simulink model "OORT"  (Simulink 7.6)
settings: Solver=ode3  SolverMode=SingleTasking  StartTime=0.0  StopTime=1.2  FixedStep=2e-5  RelTol=1e-4  AbsTol=1e-6
undefined symbols (not defined in the file or in its folder): DAB, den, elements, num
libraries: powerlib x179, powerlib_extras x6
(part 1 of 4)
settings Model: Creator=azadpour  LastModifiedBy=PC  ExtModeTrigMode=oneshot  ExtModeArmWhenConnect=off
settings SolverCC: SolverResetMethod=Robust
settings DataIOCC: LimitDataPoints=off
settings OptimizationCC: BlockReduction=off  BooleanDataType=off  InlineInvariantSignals=on  InitFltsAndDblsToZero=on
settings DebuggingCC: SaveWithDisabledLinksMsg=none  SaveWithParameterizedLinksMsg=none  CheckSSInitialOutputMsg=off  SignalResolutionControl=TryResolveAllWithWarning  SolverPrmCheckMsg=none  InheritedTsInSrcMsg=none  DiscreteInheritContinuousMsg=none  MultiTaskDSMMsg=none  MultiTaskCondExecSysMsg=none  TasksWithSamePriorityMsg=none  SigSpecEnsureSampleTimeMsg=none  IntegerOverflowMsg=none  Int32ToFloatConvMsg=none  ParameterPrecisionLossMsg=none  ParameterTunabilityLossMsg=none  UnconnectedInputMsg=none  UnconnectedOutputMsg=none  UnconnectedLineMsg=none  BusObjectLabelMismatch=none  RootOutportRequireBusObject=none  ModelReferenceDataLoggingMessage=none  StrictBusMsg=None
settings HardwareCC: TargetHWDeviceType=32-bit Generic  TargetUnknown=on  ProdEqTarget=off
settings GRTTargetCC: TargetFcnLib=ansi_tfl_tmw.mat

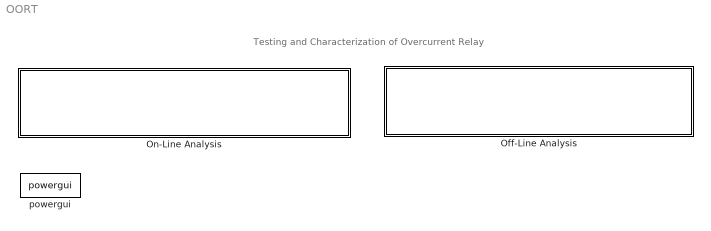
== system OORT ==
  note: Testing and Characterization of Overcurrent Relay
  Off-Line Analysis : Subsystem
      mask Type: Off-Line Analysis
      mask Display: disp('Off-Line Testing');
  On-Line Analysis : Subsystem
      mask Type: On-Line Analysis
      mask Display: disp('On-Line Testing')
  powergui : powerlib/powergui  SystemSampleTime=-1  SimulationMode=Continuous  SampleTime=0  frequency=60  SPID=off  DisableSnubberDevices=off  DisableRonSwitches=off  DisableVfSwitches=off  SwTol=0  Interpol=off  frequencyindice=60  echomessages=off  HookPort=off  DisplayEquations=off  FunctionMessages=off  EnableUseOfTLC=off  x0status=blocks  RestoreLinks=warning  ResistiveCurrentMeasurement=off  Frange=[0:2:500]  Ylog=off  Xlog=on  ShowGrid=off  save=off  variable=ZData  ZoomFFT=on  StartTime=0.0  cycles=1  DisplayStyle=1  fundamental=60  FreqAxis=off  MaxFrequency=1000  frequencyindicesteady=1  RmsSteady=1  display=off  Ts=0  methode=off

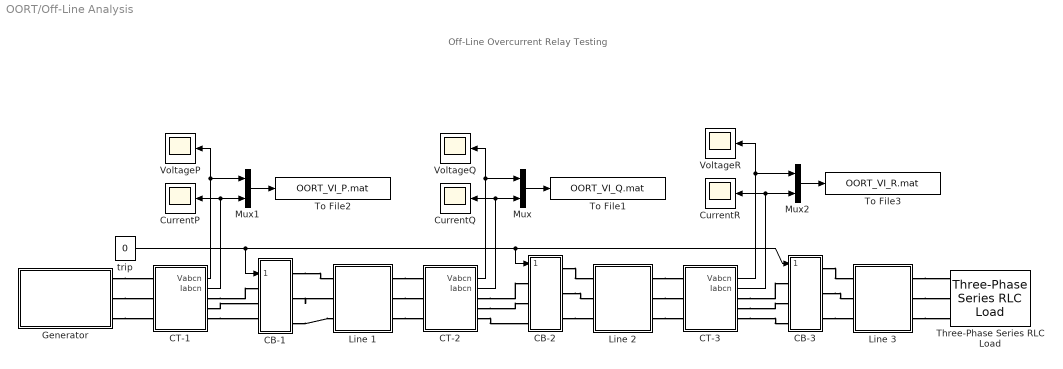
== system OORT/Off-Line Analysis ==
  note: Off-Line Overcurrent Relay Testing
  CB-1 : Subsystem  mask{t_op=0.02}
      mask prompts: t_op "Operating time [s]"
  CB-2 : Subsystem  mask{t_op=0.02}
      mask prompts: t_op "Operating time [s]"
  CB-3 : Subsystem  mask{t_op=0.02}
      mask prompts: t_op "Operating time [s]"
  CT-1 : Subsystem  mask{VT=2000, CT=100}
      mask prompts: VT "VT ratio"; CT "CT ratio"
  CT-2 : Subsystem  mask{VT=2000, CT=100}
      mask prompts: VT "VT ratio"; CT "CT ratio"
  CT-3 : Subsystem  mask{VT=2000, CT=100}
      mask prompts: VT "VT ratio"; CT "CT ratio"
  CurrentP : Scope
      settings: TickLabels=on  YMin=-8000  YMax=9000  SaveName=ScopeData12  DataFormat=Array
  CurrentQ : Scope
      settings: TickLabels=on  YMin=-8000  YMax=9000  SaveName=ScopeData13  DataFormat=Array
  CurrentR : Scope
      settings: TickLabels=on  YMin=-8000  YMax=9000  SaveName=ScopeData14  DataFormat=Array
  Generator : Subsystem  mask(3-phase inductive source - Ungrounded neutral){V=194367, Phi=0, F=60, R=3.4878, L=0.1323}
      mask prompts: V "Voltage magnitude (V) :"; Phi "Phase angle of phase A (Degrees) :"; F "Frequency (Hz) :"; R "Source resistance (Ohms):"; L "Source inductance (H) :"
      mask init:
      | a=R;b=L;c=inf;
      | short_x =[0,150];
      | short_y =[0,0];
      | 
      | resistor_x = [0 30,30,38,53,68,83,98,113,120,120,150];
      | resistor_y = [0,0,0,25,-25,25,-25,25,-25,0,0,0];
      | 
      | inductor_x = [150,173,173,174,178,184,190,197,202,205,206,204,201,201,197,196,198,201,207,214,220,225,229,229,227,224,224,220,219,221,225,230,237,243,249,252,253,251,247,247,244,243,244,248,254,260,267,272,275,276,276,300];
      | 
      | inductor_y = [0,0,1,11,19,24,25,23,17,8,-2,-12,-18,-18,-9,1,11,19,24,25,23,17,8,-2,-12,-18,-18,-9,1,11,19,24,25,23,17,8,-2,-12,-18,-18,-9,1, 11,19,24,25,23,17,8,0,0,0];
      | 
      | capacitor_x1 = [300 360 360 360];
      | capacitor_y1 = [0 0 25 -25];
      | capacitor_x2 = [390 390 390 450];
      | capacitor_y2 = [25,-25,0,0];
      | if a~=0
      | 	s1=resistor_x;
      | 	s2=resistor_y;
      | else
      | 	s1=short_x;
      | 	s2=short_y;
      | end
      | 
      | if b~=0
      | 	s3=inductor_x;
      | 	s4=inductor_y;
      | else
      | 	s3=short_x+150;
      | 	s4=short_y;
      | end
      | 
      | s5=[];
      | s6=[];
      | s7=[];
      | s8=[];
      mask Display: plot(-170,-60,360,60,s1,s2,s3,s4,s5,s6,s7,s8, [0,9,18,24,29,30,29,24,18,9,0,-9,-18,-24,-29,-30,-29,-24,-18,-9,0]*1.5-45,  [30,29,24,18,9,0,-9,-18,-24,-29,-30,-29,-24,-18,-9,0,9,18,24,29,30]*0.8,[-150,-90],[0,0],[-150,-150],[-20,20],[-165,-165],[-15,15],[-180,-180],[-10,10])
  Line 1 : Subsystem  mask(Teansmission line with fault){ff=60, rr=[0.0815 0.3666], ll=[2.1e-3 6.5e-3], cc=[31.6e-9 12.7e-9], length=40, faultLocation=0.5, faultType='C-A-G', faultR=0.01, faultTime=[9 10 11 12 13]}
      mask prompts: ff "Frequency used for R L C specification (Hz)"; rr "Resistance per unit length (Ohm/mile) [R1 R0]"; ll "Inductance per unit length (H/mile) [L1 L0]"; cc "Capacitance per unit length (F/mile) [C1 C0]"; length "Line length (mile)"; faultLocation "Fault location (p.u.) <0,1>"; faultType "Fault Type"; faultR "Fault Resistance per Phase (Ohm)"; faultTime "Fault time sequence (s) [C O C O C]"
      mask StyleString: edit,edit,edit,edit,edit,edit,popup('A-G'|'B-G'|'C-G'|'B-C'|'B-C-G'|'C-A'|'C-A-G'|'A-B-C'|'A-B-C-G'),edit,edit
  Line 2 : Subsystem  mask(Teansmission line with fault){ff=60, rr=[0.0815 0.3666], ll=[2.1e-3 6.5e-3], cc=[31.6e-9 12.7e-9], length=40, faultLocation=0.5, faultType='C-A-G', faultR=0.01, faultTime=[9 10 11 12 13]}
      mask prompts: ff "Frequency used for R L C specification (Hz)"; rr "Resistance per unit length (Ohm/mile) [R1 R0]"; ll "Inductance per unit length (H/mile) [L1 L0]"; cc "Capacitance per unit length (F/mile) [C1 C0]"; length "Line length (mile)"; faultLocation "Fault location (p.u.) <0,1>"; faultType "Fault Type"; faultR "Fault Resistance per Phase (Ohm)"; faultTime "Fault time sequence (s) [C O C O C]"
      mask StyleString: edit,edit,edit,edit,edit,edit,popup('A-G'|'B-G'|'C-G'|'B-C'|'B-C-G'|'C-A'|'C-A-G'|'A-B-C'|'A-B-C-G'),edit,edit
  Line 3 : Subsystem  mask(Teansmission line with fault){ff=60, rr=[0.0815 0.3666], ll=[2.1e-3 6.5e-3], cc=[31.6e-9 12.7e-9], length=40, faultLocation=0.9, faultType='A-B-C', faultR=0.01, faultTime=[0.02 10 11 12 13]}
      mask prompts: ff "Frequency used for R L C specification (Hz)"; rr "Resistance per unit length (Ohm/mile) [R1 R0]"; ll "Inductance per unit length (H/mile) [L1 L0]"; cc "Capacitance per unit length (F/mile) [C1 C0]"; length "Line length (mile)"; faultLocation "Fault location (p.u.) <0,1>"; faultType "Fault Type"; faultR "Fault Resistance per Phase (Ohm)"; faultTime "Fault time sequence (s) [C O C O C]"
      mask StyleString: edit,edit,edit,edit,edit,edit,popup('A-G'|'B-G'|'C-G'|'B-C'|'B-C-G'|'C-A'|'C-A-G'|'A-B-C'|'A-B-C-G'),edit,edit
  Mux : Mux  Inputs=2
  Mux1 : Mux  Inputs=2
  Mux2 : Mux  Inputs=2
  Three-Phase Series RLC Load : powerlib/Elements/Three-Phase Series RLC Load  DialogController=POWERSYS.PowerSysDialog  PhysicalDomain=powersysdomain  SubClassName=unknown  LeftPortType=p1  RightPortType=p1  LConnTagsString=A|B|C  Configuration=Y (grounded)  NominalVoltage=230e3  NominalFrequency=60  ActivePower=54e3  InductivePower=26e3  CapacitivePower=0  Measurements=None
  To File1 : ToFile  Filename=OORT_VI_Q.mat
  To File2 : ToFile  Filename=OORT_VI_P.mat
  To File3 : ToFile  Filename=OORT_VI_R.mat
  VoltageP : Scope
      settings: TickLabels=on  YMin=-8000  YMax=9000  SaveName=ScopeData21  DataFormat=Array
  VoltageQ : Scope
      settings: TickLabels=on  YMin=-8000  YMax=9000  SaveName=ScopeData22  DataFormat=Array
  VoltageR : Scope
      settings: TickLabels=on  YMin=-8000  YMax=9000  SaveName=ScopeData23  DataFormat=Array
  trip : Constant  Value=0
  wires:
  CT-2/2(Iabcn) -> CurrentQ/1, Mux/2
  CT-2/1(Vabcn) -> VoltageQ/1, Mux/1
  CT-1/2(Iabcn) -> CurrentP/1, Mux1/2
  CT-1/1(Vabcn) -> VoltageP/1, Mux1/1
  CT-3/2(Iabcn) -> CurrentR/1, Mux2/2
  CT-3/1(Vabcn) -> VoltageR/1, Mux2/1
  Mux/1 -> To File1/1
  Mux1/1 -> To File2/1
  Mux2/1 -> To File3/1
  trip/1 -> CB-1/1(Trip), CB-2/1(Trip), CB-3/1(Trip)
  connections:
  Line 1/RConn1 -- CT-2/LConn1
  Line 1/RConn2 -- CT-2/LConn2
  Line 1/RConn3 -- CT-2/LConn3
  Generator/RConn1 -- CT-1/LConn1
  Generator/RConn2 -- CT-1/LConn2
  Generator/RConn3 -- CT-1/LConn3
  CT-1/RConn1 -- CB-1/LConn1
  CT-1/RConn2 -- CB-1/LConn2
  CT-1/RConn3 -- CB-1/LConn3
  CB-1/RConn1 -- Line 1/LConn1
  CB-1/RConn2 -- Line 1/LConn2
  CB-1/RConn3 -- Line 1/LConn3
  CT-2/RConn1 -- CB-2/LConn1
  CT-2/RConn2 -- CB-2/LConn2
  CT-2/RConn3 -- CB-2/LConn3
  CB-2/RConn1 -- Line 2/LConn1
  CB-2/RConn2 -- Line 2/LConn2
  CB-2/RConn3 -- Line 2/LConn3
  Line 2/RConn1 -- CT-3/LConn1
  Line 2/RConn2 -- CT-3/LConn2
  Line 2/RConn3 -- CT-3/LConn3
  CT-3/RConn1 -- CB-3/LConn1
  CT-3/RConn2 -- CB-3/LConn2
  CT-3/RConn3 -- CB-3/LConn3
  CB-3/RConn1 -- Line 3/LConn1
  CB-3/RConn2 -- Line 3/LConn2
  CB-3/RConn3 -- Line 3/LConn3
  Line 3/RConn1 -- Three-Phase Series RLC Load/LConn1
  Line 3/RConn2 -- Three-Phase Series RLC Load/LConn2
  Line 3/RConn3 -- Three-Phase Series RLC Load/LConn3

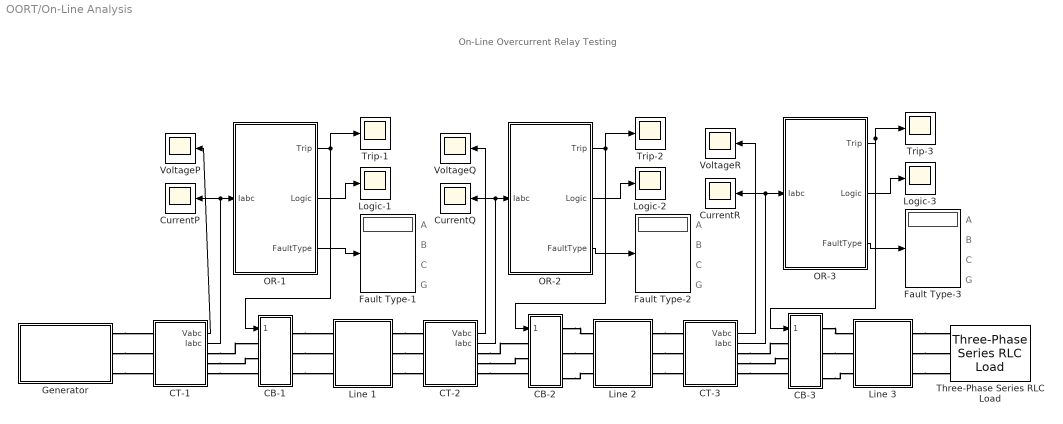
== system OORT/On-Line Analysis ==
  note: On-Line Overcurrent Relay Testing
  note: A
  note: B
  note: C
  note: G
  note: A
  note: B
  note: C
  note: G
  note: A
  note: B
  note: C
  note: G
  CB-1 : Subsystem  mask{t_op=0.02}
      mask prompts: t_op "Operating time [s]"
  CB-2 : Subsystem  mask{t_op=0.02}
      mask prompts: t_op "Operating time [s]"
  CB-3 : Subsystem  mask{t_op=0.02}
      mask prompts: t_op "Operating time [s]"
  CT-1 : Subsystem  mask{VT=2000, CT=100}
      mask prompts: VT "VT ratio"; CT "CT ratio"
  CT-2 : Subsystem  mask{VT=2000, CT=100}
      mask prompts: VT "VT ratio"; CT "CT ratio"
  CT-3 : Subsystem  mask{VT=2000, CT=100}
      mask prompts: VT "VT ratio"; CT "CT ratio"
  CurrentP : Scope
      settings: TickLabels=on  YMin=-8000  YMax=9000  SaveName=ScopeData2  DataFormat=Array
  CurrentQ : Scope
      settings: TickLabels=on  YMin=-8000  YMax=9000  DataFormat=Array
  CurrentR : Scope
      settings: TickLabels=on  YMin=-8000  YMax=9000  SaveName=ScopeData8  DataFormat=Array
  Fault Type-1 : Display
  Fault Type-2 : Display
  Fault Type-3 : Display
  Generator : Subsystem  mask(3-phase inductive source - Ungrounded neutral){V=194367, Phi=0, F=60, R=3.4878, L=0.1323}
      mask prompts: V "Voltage magnitude (V) :"; Phi "Phase angle of phase A (Degrees) :"; F "Frequency (Hz) :"; R "Source resistance (Ohms):"; L "Source inductance (H) :"
      mask init: same as OORT/Off-Line Analysis/Generator
      mask Display: plot(-170,-60,360,60,s1,s2,s3,s4,s5,s6,s7,s8, [0,9,18,24,29,30,29,24,18,9,0,-9,-18,-24,-29,-30,-29,-24,-18,-9,0]*1.5-45,  [30,29,24,18,9,0,-9,-18,-24,-29,-30,-29,-24,-18,-9,0,9,18,24,29,30]*0.8,[-150,-90],[0,0],[-150,-150],[-20,20],[-165,-165],[-15,15],[-180,-180],[-10,10])
  Line 1 : Subsystem  mask(Teansmission line with fault){ff=60, rr=[0.0815 0.3666], ll=[2.1e-3 6.5e-3], cc=[31.6e-9 12.7e-9], length=40, faultLocation=0.5, faultType='C-A-G', faultR=0.01, faultTime=[9 10 11 12 13]}
      mask prompts: ff "Frequency used for R L C specification (Hz)"; rr "Resistance per unit length (Ohm/mile) [R1 R0]"; ll "Inductance per unit length (H/mile) [L1 L0]"; cc "Capacitance per unit length (F/mile) [C1 C0]"; length "Line length (mile)"; faultLocation "Fault location (p.u.) <0,1>"; faultType "Fault Type"; faultR "Fault Resistance per Phase (Ohm)"; faultTime "Fault time sequence (s) [C O C O C]"
      mask StyleString: edit,edit,edit,edit,edit,edit,popup('A-G'|'B-G'|'C-G'|'B-C'|'B-C-G'|'C-A'|'C-A-G'|'A-B-C'|'A-B-C-G'),edit,edit
  Line 2 : Subsystem  mask(Teansmission line with fault){ff=60, rr=[0.0815 0.3666], ll=[2.1e-3 6.5e-3], cc=[31.6e-9 12.7e-9], length=40, faultLocation=0.3, faultType='B-C', faultR=0.01, faultTime=[9 10 11 12 13]}
      mask prompts: ff "Frequency used for R L C specification (Hz)"; rr "Resistance per unit length (Ohm/mile) [R1 R0]"; ll "Inductance per unit length (H/mile) [L1 L0]"; cc "Capacitance per unit length (F/mile) [C1 C0]"; length "Line length (mile)"; faultLocation "Fault location (p.u.) <0,1>"; faultType "Fault Type"; faultR "Fault Resistance per Phase (Ohm)"; faultTime "Fault time sequence (s) [C O C O C]"
      mask StyleString: edit,edit,edit,edit,edit,edit,popup('A-G'|'B-G'|'C-G'|'B-C'|'B-C-G'|'C-A'|'C-A-G'|'A-B-C'|'A-B-C-G'),edit,edit
  Line 3 : Subsystem  mask(Teansmission line with fault){ff=60, rr=[0.0815 0.3666], ll=[2.1e-3 6.5e-3], cc=[31.6e-9 12.7e-9], length=40, faultLocation=0.9, faultType='A-B-C', faultR=0.01, faultTime=[0.02 10 11 12 13]}
      mask prompts: ff "Frequency used for R L C specification (Hz)"; rr "Resistance per unit length (Ohm/mile) [R1 R0]"; ll "Inductance per unit length (H/mile) [L1 L0]"; cc "Capacitance per unit length (F/mile) [C1 C0]"; length "Line length (mile)"; faultLocation "Fault location (p.u.) <0,1>"; faultType "Fault Type"; faultR "Fault Resistance per Phase (Ohm)"; faultTime "Fault time sequence (s) [C O C O C]"
      mask StyleString: edit,edit,edit,edit,edit,edit,popup('A-G'|'B-G'|'C-G'|'B-C'|'B-C-G'|'C-A'|'C-A-G'|'A-B-C'|'A-B-C-G'),edit,edit
  Logic-1 : Scope
      settings: SaveName=ScopeData3
  Logic-2 : Scope
      settings: SaveName=ScopeData7
  Logic-3 : Scope
      settings: SaveName=ScopeData9
  OR-1 : Subsystem  mask(Overcurrent Relay){Iop=3.8, Td=1, ResCurr=0.1}
      mask prompts: Iop "Pickup Current (A):"; Td "Time Delay (s):"; ResCurr "ResidualCurrent Threshold (A):"
  OR-2 : Subsystem  mask(Overcurrent Relay){Iop=2.6, Td=0.6, ResCurr=0.1}
      mask prompts: Iop "Pickup Current (A):"; Td "Time Delay (s):"; ResCurr "ResidualCurrent Threshold (A):"
  OR-3 : Subsystem  mask(Overcurrent Relay){Iop=1.4, Td=0, ResCurr=0.1}
      mask prompts: Iop "Pickup Current (A):"; Td "Time Delay (s):"; ResCurr "ResidualCurrent Threshold (A):"
  Three-Phase Series RLC Load : powerlib/Elements/Three-Phase Series RLC Load  DialogController=POWERSYS.PowerSysDialog  PhysicalDomain=powersysdomain  SubClassName=unknown  LeftPortType=p1  RightPortType=p1  LConnTagsString=A|B|C  Configuration=Y (grounded)  NominalVoltage=230e3  NominalFrequency=60  ActivePower=54e3  InductivePower=26e3  CapacitivePower=0  Measurements=None
  Trip-1 : Scope
      settings: YMin=-0.2  YMax=1.2  SaveName=ScopeData4
  Trip-2 : Scope
      settings: YMin=-0.2  YMax=1.2  SaveName=ScopeData6
  Trip-3 : Scope
      settings: TimeRange=0.2  YMin=-0.2  YMax=1.2  SaveName=ScopeData10
  VoltageP : Scope
      settings: TickLabels=on  YMin=-8000  YMax=9000  SaveName=ScopeData5  DataFormat=Array
  VoltageQ : Scope
      settings: TickLabels=on  YMin=-8000  YMax=9000  DataFormat=Array
  VoltageR : Scope
      settings: TickLabels=on  YMin=-8000  YMax=9000  SaveName=ScopeData11  DataFormat=Array
  wires:
  CT-2/2(Iabc) -> CurrentQ/1, OR-2/1(Iabc)
  CT-2/1(Vabc) -> VoltageQ/1
  OR-2/1(Trip) -> Trip-2/1, CB-2/1(Trip)
  OR-2/2(Logic) -> Logic-2/1
  OR-2/3(FaultType) -> Fault Type-2/1
  OR-1/1(Trip) -> Trip-1/1, CB-1/1(Trip)
  OR-1/2(Logic) -> Logic-1/1
  CT-1/2(Iabc) -> OR-1/1(Iabc), CurrentP/1
  CT-1/1(Vabc) -> VoltageP/1
  OR-3/1(Trip) -> Trip-3/1, CB-3/1(Trip)
  OR-3/2(Logic) -> Logic-3/1
  OR-3/3(FaultType) -> Fault Type-3/1
  CT-3/2(Iabc) -> CurrentR/1, OR-3/1(Iabc)
  CT-3/1(Vabc) -> VoltageR/1
  OR-1/3(FaultType) -> Fault Type-1/1
  connections:
  Line 1/RConn1 -- CT-2/LConn1
  Line 1/RConn2 -- CT-2/LConn2
  Line 1/RConn3 -- CT-2/LConn3
  Generator/RConn1 -- CT-1/LConn1
  Generator/RConn2 -- CT-1/LConn2
  Generator/RConn3 -- CT-1/LConn3
  CT-1/RConn1 -- CB-1/LConn1
  CT-1/RConn2 -- CB-1/LConn2
  CT-1/RConn3 -- CB-1/LConn3
  CB-1/RConn1 -- Line 1/LConn1
  CB-1/RConn2 -- Line 1/LConn2
  CB-1/RConn3 -- Line 1/LConn3
  CT-2/RConn1 -- CB-2/LConn1
  CT-2/RConn2 -- CB-2/LConn2
  CT-2/RConn3 -- CB-2/LConn3
  CB-2/RConn1 -- Line 2/LConn1
  CB-2/RConn2 -- Line 2/LConn2
  CB-2/RConn3 -- Line 2/LConn3
  Line 2/RConn1 -- CT-3/LConn1
  Line 2/RConn2 -- CT-3/LConn2
  Line 2/RConn3 -- CT-3/LConn3
  CT-3/RConn1 -- CB-3/LConn1
  CT-3/RConn2 -- CB-3/LConn2
  CT-3/RConn3 -- CB-3/LConn3
  CB-3/RConn1 -- Line 3/LConn1
  CB-3/RConn2 -- Line 3/LConn2
  CB-3/RConn3 -- Line 3/LConn3
  Line 3/RConn1 -- Three-Phase Series RLC Load/LConn1
  Line 3/RConn2 -- Three-Phase Series RLC Load/LConn2
  Line 3/RConn3 -- Three-Phase Series RLC Load/LConn3

== system OORT/Off-Line Analysis/CB-1 ==
  Trip : Inport
  BreakerA : powerlib/Elements/Breaker  DialogController=POWERSYS.PowerSysDialog  SystemSampleTime=-1  BreakerResistance=0.01  InitialState=1  SnubberResistance=1e6  SnubberCapacitance=inf  SwitchingTimes="[ 1/60  5/60 ]"  External=on  Measurements=None  MoreParameters=off  NoBreakLoop=off
  BreakerB : powerlib/Elements/Breaker  DialogController=POWERSYS.PowerSysDialog  SystemSampleTime=-1  BreakerResistance=0.01  InitialState=1  SnubberResistance=1e6  SnubberCapacitance=inf  SwitchingTimes="[ 1/60  5/60 ]"  External=on  Measurements=None  MoreParameters=off  NoBreakLoop=off
  BreakerC : powerlib/Elements/Breaker  DialogController=POWERSYS.PowerSysDialog  SystemSampleTime=-1  BreakerResistance=0.01  InitialState=1  SnubberResistance=1e6  SnubberCapacitance=inf  SwitchingTimes="[ 1/60  5/60 ]"  External=on  Measurements=None  MoreParameters=off  NoBreakLoop=off
  NOT : Logic  Operator=NOT  Inputs=1
  Series RLC Branch1 : powerlib/Elements/Series RLC Branch  DialogController=POWERSYS.PowerSysDialog  PhysicalDomain=powersysdomain  SubClassName=unknown  LeftPortType=p1  RightPortType=p1  LConnTagsString=__new0  RConnTagsString=__new0  BranchType=R  Resistance=1e6  Inductance=1.0  SetiL0=off  InitialCurrent=0  Capacitance=1.0  Setx0=off  InitialVoltage=0  Measurements=None
  Series RLC Branch2 : powerlib/Elements/Series RLC Branch  DialogController=POWERSYS.PowerSysDialog  PhysicalDomain=powersysdomain  SubClassName=unknown  LeftPortType=p1  RightPortType=p1  LConnTagsString=__new0  RConnTagsString=__new0  BranchType=R  Resistance=1e6  Inductance=1.0  SetiL0=off  InitialCurrent=0  Capacitance=1.0  Setx0=off  InitialVoltage=0  Measurements=None
  Series RLC Branch3 : powerlib/Elements/Series RLC Branch  DialogController=POWERSYS.PowerSysDialog  PhysicalDomain=powersysdomain  SubClassName=unknown  LeftPortType=p1  RightPortType=p1  LConnTagsString=__new0  RConnTagsString=__new0  BranchType=R  Resistance=1e6  Inductance=1.0  SetiL0=off  InitialCurrent=0  Capacitance=1.0  Setx0=off  InitialVoltage=0  Measurements=None
  Transport Delay : TransportDelay  DelayTime=t_op+0.001  BufferSize=10240
  A1 : PMIOPort  Tag=PMCPort  Port=1  Side=Left
  B1 : PMIOPort  Tag=PMCPort  Port=2  Side=Left
  C1 : PMIOPort  Tag=PMCPort  Port=3  Side=Left
  A2 : PMIOPort  Tag=PMCPort  Port=4  Side=Right
  B2 : PMIOPort  Tag=PMCPort  Port=5  Side=Right
  C2 : PMIOPort  Tag=PMCPort  Port=6  Side=Right
  wires:
  NOT/1 -> BreakerA/1, BreakerB/1, BreakerC/1
  Transport Delay/1 -> NOT/1
  Trip/1 -> Transport Delay/1
  connections:
  A2/RConn1 -- BreakerA/RConn1 -- Series RLC Branch1/RConn1
  B2/RConn1 -- BreakerB/RConn1 -- Series RLC Branch2/RConn1
  C2/RConn1 -- BreakerC/RConn1 -- Series RLC Branch3/RConn1
  A1/RConn1 -- BreakerA/LConn1 -- Series RLC Branch1/LConn1
  B1/RConn1 -- BreakerB/LConn1 -- Series RLC Branch2/LConn1
  C1/RConn1 -- BreakerC/LConn1 -- Series RLC Branch3/LConn1

== system OORT/Off-Line Analysis/CB-2 ==
  Trip : Inport
  BreakerA : powerlib/Elements/Breaker  DialogController=POWERSYS.PowerSysDialog  SystemSampleTime=-1  BreakerResistance=0.01  InitialState=1  SnubberResistance=1e6  SnubberCapacitance=inf  SwitchingTimes="[ 1/60  5/60 ]"  External=on  Measurements=None  MoreParameters=off  NoBreakLoop=off
  BreakerB : powerlib/Elements/Breaker  DialogController=POWERSYS.PowerSysDialog  SystemSampleTime=-1  BreakerResistance=0.01  InitialState=1  SnubberResistance=1e6  SnubberCapacitance=inf  SwitchingTimes="[ 1/60  5/60 ]"  External=on  Measurements=None  MoreParameters=off  NoBreakLoop=off
  BreakerC : powerlib/Elements/Breaker  DialogController=POWERSYS.PowerSysDialog  SystemSampleTime=-1  BreakerResistance=0.01  InitialState=1  SnubberResistance=1e6  SnubberCapacitance=inf  SwitchingTimes="[ 1/60  5/60 ]"  External=on  Measurements=None  MoreParameters=off  NoBreakLoop=off
  NOT : Logic  Operator=NOT  Inputs=1
  Series RLC Branch1 : powerlib/Elements/Series RLC Branch  DialogController=POWERSYS.PowerSysDialog  PhysicalDomain=powersysdomain  SubClassName=unknown  LeftPortType=p1  RightPortType=p1  LConnTagsString=__new0  RConnTagsString=__new0  BranchType=R  Resistance=1e6  Inductance=1.0  SetiL0=off  InitialCurrent=0  Capacitance=1.0  Setx0=off  InitialVoltage=0  Measurements=None
  Series RLC Branch2 : powerlib/Elements/Series RLC Branch  DialogController=POWERSYS.PowerSysDialog  PhysicalDomain=powersysdomain  SubClassName=unknown  LeftPortType=p1  RightPortType=p1  LConnTagsString=__new0  RConnTagsString=__new0  BranchType=R  Resistance=1e6  Inductance=1.0  SetiL0=off  InitialCurrent=0  Capacitance=1.0  Setx0=off  InitialVoltage=0  Measurements=None
  Series RLC Branch3 : powerlib/Elements/Series RLC Branch  DialogController=POWERSYS.PowerSysDialog  PhysicalDomain=powersysdomain  SubClassName=unknown  LeftPortType=p1  RightPortType=p1  LConnTagsString=__new0  RConnTagsString=__new0  BranchType=R  Resistance=1e6  Inductance=1.0  SetiL0=off  InitialCurrent=0  Capacitance=1.0  Setx0=off  InitialVoltage=0  Measurements=None
  Transport Delay : TransportDelay  DelayTime=t_op+0.001  BufferSize=10240
  A1 : PMIOPort  Tag=PMCPort  Port=1  Side=Left
  B1 : PMIOPort  Tag=PMCPort  Port=2  Side=Left
  C1 : PMIOPort  Tag=PMCPort  Port=3  Side=Left
  A2 : PMIOPort  Tag=PMCPort  Port=4  Side=Right
  B2 : PMIOPort  Tag=PMCPort  Port=5  Side=Right
  C2 : PMIOPort  Tag=PMCPort  Port=6  Side=Right
  wires:
  Trip/1 -> Transport Delay/1
  Transport Delay/1 -> NOT/1
  NOT/1 -> BreakerC/1, BreakerB/1, BreakerA/1
  connections:
  Series RLC Branch3/LConn1 -- BreakerC/LConn1 -- C1/RConn1
  Series RLC Branch2/LConn1 -- BreakerB/LConn1 -- B1/RConn1
  Series RLC Branch1/LConn1 -- BreakerA/LConn1 -- A1/RConn1
  Series RLC Branch3/RConn1 -- BreakerC/RConn1 -- C2/RConn1
  Series RLC Branch2/RConn1 -- BreakerB/RConn1 -- B2/RConn1
  Series RLC Branch1/RConn1 -- BreakerA/RConn1 -- A2/RConn1

== system OORT/Off-Line Analysis/CB-3 ==
  Trip : Inport
  BreakerA : powerlib/Elements/Breaker  DialogController=POWERSYS.PowerSysDialog  SystemSampleTime=-1  BreakerResistance=0.01  InitialState=1  SnubberResistance=1e6  SnubberCapacitance=inf  SwitchingTimes="[ 1/60  5/60 ]"  External=on  Measurements=None  MoreParameters=off  NoBreakLoop=off
  BreakerB : powerlib/Elements/Breaker  DialogController=POWERSYS.PowerSysDialog  SystemSampleTime=-1  BreakerResistance=0.01  InitialState=1  SnubberResistance=1e6  SnubberCapacitance=inf  SwitchingTimes="[ 1/60  5/60 ]"  External=on  Measurements=None  MoreParameters=off  NoBreakLoop=off
  BreakerC : powerlib/Elements/Breaker  DialogController=POWERSYS.PowerSysDialog  SystemSampleTime=-1  BreakerResistance=0.01  InitialState=1  SnubberResistance=1e6  SnubberCapacitance=inf  SwitchingTimes="[ 1/60  5/60 ]"  External=on  Measurements=None  MoreParameters=off  NoBreakLoop=off
  NOT : Logic  Operator=NOT  Inputs=1
  Series RLC Branch1 : powerlib/Elements/Series RLC Branch  DialogController=POWERSYS.PowerSysDialog  PhysicalDomain=powersysdomain  SubClassName=unknown  LeftPortType=p1  RightPortType=p1  LConnTagsString=__new0  RConnTagsString=__new0  BranchType=R  Resistance=1e6  Inductance=1.0  SetiL0=off  InitialCurrent=0  Capacitance=1.0  Setx0=off  InitialVoltage=0  Measurements=None
  Series RLC Branch2 : powerlib/Elements/Series RLC Branch  DialogController=POWERSYS.PowerSysDialog  PhysicalDomain=powersysdomain  SubClassName=unknown  LeftPortType=p1  RightPortType=p1  LConnTagsString=__new0  RConnTagsString=__new0  BranchType=R  Resistance=1e6  Inductance=1.0  SetiL0=off  InitialCurrent=0  Capacitance=1.0  Setx0=off  InitialVoltage=0  Measurements=None
  Series RLC Branch3 : powerlib/Elements/Series RLC Branch  DialogController=POWERSYS.PowerSysDialog  PhysicalDomain=powersysdomain  SubClassName=unknown  LeftPortType=p1  RightPortType=p1  LConnTagsString=__new0  RConnTagsString=__new0  BranchType=R  Resistance=1e6  Inductance=1.0  SetiL0=off  InitialCurrent=0  Capacitance=1.0  Setx0=off  InitialVoltage=0  Measurements=None
  Transport Delay : TransportDelay  DelayTime=t_op+0.001  BufferSize=10240
  A1 : PMIOPort  Tag=PMCPort  Port=1  Side=Left
  B1 : PMIOPort  Tag=PMCPort  Port=2  Side=Left
  C1 : PMIOPort  Tag=PMCPort  Port=3  Side=Left
  A2 : PMIOPort  Tag=PMCPort  Port=4  Side=Right
  B2 : PMIOPort  Tag=PMCPort  Port=5  Side=Right
  C2 : PMIOPort  Tag=PMCPort  Port=6  Side=Right
  wires:
  NOT/1 -> BreakerA/1, BreakerB/1, BreakerC/1
  Transport Delay/1 -> NOT/1
  Trip/1 -> Transport Delay/1
  connections:
  A2/RConn1 -- BreakerA/RConn1 -- Series RLC Branch1/RConn1
  B2/RConn1 -- BreakerB/RConn1 -- Series RLC Branch2/RConn1
  C2/RConn1 -- BreakerC/RConn1 -- Series RLC Branch3/RConn1
  A1/RConn1 -- BreakerA/LConn1 -- Series RLC Branch1/LConn1
  B1/RConn1 -- BreakerB/LConn1 -- Series RLC Branch2/LConn1
  C1/RConn1 -- BreakerC/LConn1 -- Series RLC Branch3/LConn1

== system OORT/Off-Line Analysis/CT-1 ==
  Add : Sum  Inputs=+++
  Add1 : Sum  Inputs=+++
  CT-ratio : Gain  Gain=1/CT  SaturateOnIntegerOverflow=on  OutDataTypeStr=Inherit: Same as input  ParamDataTypeStr=Inherit: Same as input
  Ground : powerlib/Elements/Ground  DialogController=POWERSYS.PowerSysDialog  PhysicalDomain=powersysdomain  SubClassName=unknown  LeftPortType=p1  RightPortType=p1  LConnTagsString=a
  IA : powerlib/Measurements/Current Measurement  DialogController=POWERSYS.PowerSysDialog  SystemSampleTime=-1  PhasorSimulation=off  OutputType=Complex  PSBequivalent=0
  IB : powerlib/Measurements/Current Measurement  DialogController=POWERSYS.PowerSysDialog  SystemSampleTime=-1  PhasorSimulation=off  OutputType=Complex  PSBequivalent=0
  IC : powerlib/Measurements/Current Measurement  DialogController=POWERSYS.PowerSysDialog  SystemSampleTime=-1  PhasorSimulation=off  OutputType=Complex  PSBequivalent=0
  Mux : Mux
  Mux1 : Mux
  VA : powerlib/Measurements/Voltage Measurement  DialogController=POWERSYS.PowerSysDialog  SystemSampleTime=-1  PhasorSimulation=off  OutputType=Complex  PSBequivalent=0
  VB : powerlib/Measurements/Voltage Measurement  DialogController=POWERSYS.PowerSysDialog  SystemSampleTime=-1  PhasorSimulation=off  OutputType=Complex  PSBequivalent=0
  VC : powerlib/Measurements/Voltage Measurement  DialogController=POWERSYS.PowerSysDialog  SystemSampleTime=-1  PhasorSimulation=off  OutputType=Complex  PSBequivalent=0
  VT-ratio : Gain  Gain=1/VT  SaturateOnIntegerOverflow=on  OutDataTypeStr=Inherit: Same as input  ParamDataTypeStr=Inherit: Same as input
  A1 : PMIOPort  Tag=PMCPort  Port=1  Side=Left
  B1 : PMIOPort  Tag=PMCPort  Port=2  Side=Left
  C1 : PMIOPort  Tag=PMCPort  Port=3  Side=Left
  A2 : PMIOPort  Tag=PMCPort  Port=4  Side=Right
  B2 : PMIOPort  Tag=PMCPort  Port=5  Side=Right
  C2 : PMIOPort  Tag=PMCPort  Port=6  Side=Right
  Vabcn : Outport  InitialOutput=0
  Iabcn : Outport  Port=2  InitialOutput=0
  wires:
  Mux1/1 -> VT-ratio/1
  VT-ratio/1 -> Vabcn/1
  Mux/1 -> CT-ratio/1
  CT-ratio/1 -> Iabcn/1
  IA/1 -> Mux/1, Add/1
  IB/1 -> Mux/2, Add/2
  IC/1 -> Mux/3, Add/3
  Add/1 -> Mux/4
  VA/1 -> Mux1/1, Add1/1
  VB/1 -> Mux1/2, Add1/2
  VC/1 -> Mux1/3, Add1/3
  Add1/1 -> Mux1/4
  connections:
  VA/LConn2 -- VB/LConn2 -- Ground/LConn1 -- VC/LConn2
  A1/RConn1 -- IA/LConn1 -- VA/LConn1
  B1/RConn1 -- IB/LConn1 -- VB/LConn1
  C1/RConn1 -- IC/LConn1 -- VC/LConn1
  A2/RConn1 -- IA/RConn1
  IB/RConn1 -- B2/RConn1
  IC/RConn1 -- C2/RConn1

== system OORT/Off-Line Analysis/CT-2 ==
  Add : Sum  Inputs=+++
  Add1 : Sum  Inputs=+++
  CT-ratio : Gain  Gain=1/CT  SaturateOnIntegerOverflow=on  OutDataTypeStr=Inherit: Same as input  ParamDataTypeStr=Inherit: Same as input
  Ground : powerlib/Elements/Ground  DialogController=POWERSYS.PowerSysDialog  PhysicalDomain=powersysdomain  SubClassName=unknown  LeftPortType=p1  RightPortType=p1  LConnTagsString=a
  IA : powerlib/Measurements/Current Measurement  DialogController=POWERSYS.PowerSysDialog  SystemSampleTime=-1  PhasorSimulation=off  OutputType=Complex  PSBequivalent=0
  IB : powerlib/Measurements/Current Measurement  DialogController=POWERSYS.PowerSysDialog  SystemSampleTime=-1  PhasorSimulation=off  OutputType=Complex  PSBequivalent=0
  IC : powerlib/Measurements/Current Measurement  DialogController=POWERSYS.PowerSysDialog  SystemSampleTime=-1  PhasorSimulation=off  OutputType=Complex  PSBequivalent=0
  Mux : Mux
  Mux1 : Mux
  VA : powerlib/Measurements/Voltage Measurement  DialogController=POWERSYS.PowerSysDialog  SystemSampleTime=-1  PhasorSimulation=off  OutputType=Complex  PSBequivalent=0
  VB : powerlib/Measurements/Voltage Measurement  DialogController=POWERSYS.PowerSysDialog  SystemSampleTime=-1  PhasorSimulation=off  OutputType=Complex  PSBequivalent=0
  VC : powerlib/Measurements/Voltage Measurement  DialogController=POWERSYS.PowerSysDialog  SystemSampleTime=-1  PhasorSimulation=off  OutputType=Complex  PSBequivalent=0
  VT-ratio : Gain  Gain=1/VT  SaturateOnIntegerOverflow=on  OutDataTypeStr=Inherit: Same as input  ParamDataTypeStr=Inherit: Same as input
  A1 : PMIOPort  Tag=PMCPort  Port=1  Side=Left
  B1 : PMIOPort  Tag=PMCPort  Port=2  Side=Left
  C1 : PMIOPort  Tag=PMCPort  Port=3  Side=Left
  A2 : PMIOPort  Tag=PMCPort  Port=4  Side=Right
  B2 : PMIOPort  Tag=PMCPort  Port=5  Side=Right
  C2 : PMIOPort  Tag=PMCPort  Port=6  Side=Right
  Vabcn : Outport  InitialOutput=0
  Iabcn : Outport  Port=2  InitialOutput=0
  wires:
  Mux1/1 -> VT-ratio/1
  VT-ratio/1 -> Vabcn/1
  Mux/1 -> CT-ratio/1
  CT-ratio/1 -> Iabcn/1
  IA/1 -> Mux/1, Add/1
  IB/1 -> Mux/2, Add/2
  IC/1 -> Mux/3, Add/3
  Add/1 -> Mux/4
  VA/1 -> Mux1/1, Add1/1
  VB/1 -> Mux1/2, Add1/2
  VC/1 -> Mux1/3, Add1/3
  Add1/1 -> Mux1/4
  connections:
  VA/LConn2 -- VB/LConn2 -- Ground/LConn1 -- VC/LConn2
  A1/RConn1 -- IA/LConn1 -- VA/LConn1
  B1/RConn1 -- IB/LConn1 -- VB/LConn1
  C1/RConn1 -- IC/LConn1 -- VC/LConn1
  A2/RConn1 -- IA/RConn1
  IB/RConn1 -- B2/RConn1
  IC/RConn1 -- C2/RConn1

== system OORT/Off-Line Analysis/CT-3 ==
  Add : Sum  Inputs=+++
  Add1 : Sum  Inputs=+++
  CT-ratio : Gain  Gain=1/CT  SaturateOnIntegerOverflow=on  OutDataTypeStr=Inherit: Same as input  ParamDataTypeStr=Inherit: Same as input
  Ground : powerlib/Elements/Ground  DialogController=POWERSYS.PowerSysDialog  PhysicalDomain=powersysdomain  SubClassName=unknown  LeftPortType=p1  RightPortType=p1  LConnTagsString=a
  IA : powerlib/Measurements/Current Measurement  DialogController=POWERSYS.PowerSysDialog  SystemSampleTime=-1  PhasorSimulation=off  OutputType=Complex  PSBequivalent=0
  IB : powerlib/Measurements/Current Measurement  DialogController=POWERSYS.PowerSysDialog  SystemSampleTime=-1  PhasorSimulation=off  OutputType=Complex  PSBequivalent=0
  IC : powerlib/Measurements/Current Measurement  DialogController=POWERSYS.PowerSysDialog  SystemSampleTime=-1  PhasorSimulation=off  OutputType=Complex  PSBequivalent=0
  Mux : Mux
  Mux1 : Mux
  VA : powerlib/Measurements/Voltage Measurement  DialogController=POWERSYS.PowerSysDialog  SystemSampleTime=-1  PhasorSimulation=off  OutputType=Complex  PSBequivalent=0
  VB : powerlib/Measurements/Voltage Measurement  DialogController=POWERSYS.PowerSysDialog  SystemSampleTime=-1  PhasorSimulation=off  OutputType=Complex  PSBequivalent=0
  VC : powerlib/Measurements/Voltage Measurement  DialogController=POWERSYS.PowerSysDialog  SystemSampleTime=-1  PhasorSimulation=off  OutputType=Complex  PSBequivalent=0
  VT-ratio : Gain  Gain=1/VT  SaturateOnIntegerOverflow=on  OutDataTypeStr=Inherit: Same as input  ParamDataTypeStr=Inherit: Same as input
  A1 : PMIOPort  Tag=PMCPort  Port=1  Side=Left
  B1 : PMIOPort  Tag=PMCPort  Port=2  Side=Left
  C1 : PMIOPort  Tag=PMCPort  Port=3  Side=Left
  A2 : PMIOPort  Tag=PMCPort  Port=4  Side=Right
  B2 : PMIOPort  Tag=PMCPort  Port=5  Side=Right
  C2 : PMIOPort  Tag=PMCPort  Port=6  Side=Right
  Vabcn : Outport  InitialOutput=0
  Iabcn : Outport  Port=2  InitialOutput=0
  wires:
  Mux1/1 -> VT-ratio/1
  VT-ratio/1 -> Vabcn/1
  Mux/1 -> CT-ratio/1
  CT-ratio/1 -> Iabcn/1
  IA/1 -> Mux/1, Add/1
  IB/1 -> Mux/2, Add/2
  IC/1 -> Mux/3, Add/3
  Add/1 -> Mux/4
  VA/1 -> Mux1/1, Add1/1
  VB/1 -> Mux1/2, Add1/2
  VC/1 -> Mux1/3, Add1/3
  Add1/1 -> Mux1/4
  connections:
  VA/LConn2 -- VB/LConn2 -- Ground/LConn1 -- VC/LConn2
  A1/RConn1 -- IA/LConn1 -- VA/LConn1
  B1/RConn1 -- IB/LConn1 -- VB/LConn1
  C1/RConn1 -- IC/LConn1 -- VC/LConn1
  A2/RConn1 -- IA/RConn1
  IB/RConn1 -- B2/RConn1
  IC/RConn1 -- C2/RConn1

== system OORT/Off-Line Analysis/Generator ==
  Ground : powerlib/Elements/Ground  DialogController=POWERSYS.PowerSysDialog  PhysicalDomain=powersysdomain  SubClassName=unknown  LeftPortType=p1  RightPortType=p1  LConnTagsString=a
  RA : powerlib/Elements/Series RLC Branch  DialogController=POWERSYS.PowerSysDialog  PhysicalDomain=powersysdomain  SubClassName=unknown  LeftPortType=p1  RightPortType=p1  LConnTagsString=__new0  RConnTagsString=__new0  BranchType=RL  Resistance=R  Inductance=L  SetiL0=off  InitialCurrent=0  Capacitance=1.0  Setx0=off  InitialVoltage=0  Measurements=None
  RB : powerlib/Elements/Series RLC Branch  DialogController=POWERSYS.PowerSysDialog  PhysicalDomain=powersysdomain  SubClassName=unknown  LeftPortType=p1  RightPortType=p1  LConnTagsString=__new0  RConnTagsString=__new0  BranchType=RL  Resistance=R  Inductance=L  SetiL0=off  InitialCurrent=0  Capacitance=1.0  Setx0=off  InitialVoltage=0  Measurements=None
  RC : powerlib/Elements/Series RLC Branch  DialogController=POWERSYS.PowerSysDialog  PhysicalDomain=powersysdomain  SubClassName=unknown  LeftPortType=p1  RightPortType=p1  LConnTagsString=__new0  RConnTagsString=__new0  BranchType=RL  Resistance=R  Inductance=L  SetiL0=off  InitialCurrent=0  Capacitance=1.0  Setx0=off  InitialVoltage=0  Measurements=None
  VA : powerlib/Electrical Sources/AC Voltage Source  DialogController=POWERSYS.PowerSysDialog  SystemSampleTime=-1  Amplitude=V  Phase=Phi  Frequency=F  SampleTime=0  Measurements=None
  VB : powerlib/Electrical Sources/AC Voltage Source  DialogController=POWERSYS.PowerSysDialog  SystemSampleTime=-1  Amplitude=V  Phase=Phi-120  Frequency=F  SampleTime=0  Measurements=None
  VC : powerlib/Electrical Sources/AC Voltage Source  DialogController=POWERSYS.PowerSysDialog  SystemSampleTime=-1  Amplitude=V  Phase=Phi+120  Frequency=F  SampleTime=0  Measurements=None
  A : PMIOPort  Tag=PMCPort  Port=1  Side=Right
  B : PMIOPort  Tag=PMCPort  Port=2  Side=Right
  C : PMIOPort  Tag=PMCPort  Port=3  Side=Right
  connections:
  VC/LConn1 -- VA/LConn1 -- Ground/LConn1 -- VB/LConn1
  VA/RConn1 -- RA/LConn1
  VB/RConn1 -- RB/LConn1
  VC/RConn1 -- RC/LConn1
  RA/RConn1 -- A/RConn1
  RB/RConn1 -- B/RConn1
  RC/RConn1 -- C/RConn1

== system OORT/Off-Line Analysis/Line 1 ==
  Fault : Subsystem
  Fault Selector : Subsystem
  Line1 : powerlib/Elements/Distributed Parameters Line  DialogController=POWERSYS.PowerSysDialog  SystemSampleTime=-1  Phases=3  Frequency=ff  Resistance=rr  Inductance=ll  Capacitance=cc  Length=length*faultLocation  x1=[0 1.49951639527058e-009 108943.556003176 -232502.11164661;3.63428122191995e-005 1.48829541068799e-009 112118.723558778 -230987.709937781;7.26856244383991e-005 1.47679505489678e-009 115272.845061907 -229429.949017306;0.000109028436657599 1.46501748665406e-009 118405.328445469 -227829.121295919;0.000145371248876798 1.4529649167531e-009 121515.585704112 -226185.527268516;0.000181714061095998 1.44063960760832e-009 124603.033004597 -224499.475457751]  x2=[0 3.09525318916024e-009 109471.998953536 -238249.17618028;3.63428122191995e-005 3.07688937942974e-009 112725.854504731 -236726.995147666;7.26856244383991e-005 3.05794800001883e-009 115958.550037565 -235160.377569544;0.000109028436657599 3.03843260645553e-009 119169.478735643 -233549.617519148;0.000145371248876798 3.01834686201734e-009 122358.037868467 -231895.017355793;0.000181714061095998 2.99769453704357e-009 125523.628904582 -230196.887668121]  x3=[0 1.72726847558779e-011 38.12150299182 -980.372207781168;3.63428122191995e-005 1.76592058881694e-011 51.5495034935516 -979.757910644077;7.26856244383991e-005 1.80424121720399e-011 64.9678275244755 -978.959700992248;0.000109028436657599 1.84222316749939e-011 78.3739563014419 -977.977728659371;0.000145371248876798 1.87985931002762e-011 91.7653733304992 -976.812177973636;0.000181714061095998 1.9171425800255e-011 105.13956487927 -975.463267723129]  x4=[0 -9.70588302061896e-012 749.21057665801 -863.037321893415;3.63428122191995e-005 -1.01552180033893e-011 760.964291823719 -852.691769472656;7.26856244383991e-005 -1.06026467278275e-011 772.575164706641 -842.186156402305;0.000109028436657599 -1.10480852061023e-011 784.041015804261 -831.522454714125;0.000145371248876798 -1.14914498239764e-011 795.359692836422 -820.702666115038;0.000181714061095998 -1.19326573565009e-011 806.529071149336 -809.728821611387]  x5=0.000181714061095998  Measurements=None
  Line2 : powerlib/Elements/Distributed Parameters Line  DialogController=POWERSYS.PowerSysDialog  SystemSampleTime=-1  Phases=3  Frequency=ff  Resistance=rr  Inductance=ll  Capacitance=cc  Length=length*(1-faultLocation)  x1=[0 3.09525318916024e-009 109471.998953536 -238249.17618028;3.63428122191995e-005 3.07688937942974e-009 112725.854504731 -236726.995147666;7.26856244383991e-005 3.05794800001883e-009 115958.550037565 -235160.377569544;0.000109028436657599 3.03843260645553e-009 119169.478735643 -233549.617519148;0.000145371248876798 3.01834686201734e-009 122358.037868467 -231895.017355793;0.000181714061095998 2.99769453704357e-009 125523.628904582 -230196.887668121]  x2=[0 4.44909370376933e-009 110078.823778532 -242919.448506557;3.63428122191995e-005 4.41948556272246e-009 113396.607389142 -241388.515343684;7.26856244383991e-005 4.38904783030933e-009 116693.10507289 -239812.270611081;0.000109028436657599 4.35778622006372e-009 119967.698036939 -238191.010189119;0.000145371248876798 4.32570660017132e-009 123219.771600231 -236525.038408161;0.000181714061095998 4.29281499236822e-009 126448.715308879 -234814.667991438]  x3=[0 2.43379003255816e-011 107.105509769641 -1000.60455997175;3.63428122191995e-005 2.46373020069737e-011 120.80422881574 -999.043249293801;7.26856244383991e-005 2.49320789661571e-011 134.480271434049 -997.294406007728;0.000109028436657599 2.52221758698998e-011 148.131070464495 -995.358358392758;0.000145371248876798 2.55075382634731e-011 161.754063485534 -993.235469868653;0.000181714061095998 2.57881125808739e-011 175.346693295149 -990.92613892749]  x4=[0 -1.53284615492848e-011 683.372100240462 -883.158801021893;3.63428122191995e-005 -1.57072216440729e-011 695.407668847988 -873.713379385306;7.26856244383991e-005 -1.60830333017004e-011 707.312700950774 -864.103951086444;0.000109028436657599 -1.64558259777336e-011 719.084961829032 -854.33231993225;0.000145371248876798 -1.68255296944383e-011 730.722241685749 -844.400320177126;0.000181714061095998 -1.7192075053916e-011 742.222356061501 -834.309816178614]  x5=0.000181714061095998  Measurements=None
  Timer : powerlib_extras/Control  Blocks/Timer  DialogController=POWERSYS.PowerSysDialog  SystemSampleTime=-1  t=[0 faultTime]  e=[0 1 0 1 0 1]
  A1 : PMIOPort  Tag=PMCPort  Port=1  Side=Left
  B1 : PMIOPort  Tag=PMCPort  Port=2  Side=Left
  C1 : PMIOPort  Tag=PMCPort  Port=3  Side=Left
  A2 : PMIOPort  Tag=PMCPort  Port=4  Side=Right
  B2 : PMIOPort  Tag=PMCPort  Port=5  Side=Right
  C2 : PMIOPort  Tag=PMCPort  Port=6  Side=Right
  wires:
  Timer/1 -> Fault/5(Tfault)
  Fault Selector/4(faultG) -> Fault/4(faultG)
  Fault Selector/3(faultC) -> Fault/3(faultC)
  Fault Selector/2(faultB) -> Fault/2(faultB)
  Fault Selector/1(faultA) -> Fault/1(faultA)
  connections:
  Line2/RConn3 -- C2/RConn1
  Line2/RConn2 -- B2/RConn1
  Line2/RConn1 -- A2/RConn1
  C1/RConn1 -- Line1/LConn3
  B1/RConn1 -- Line1/LConn2
  A1/RConn1 -- Line1/LConn1
  Fault/LConn3 -- Line1/RConn3 -- Line2/LConn3
  Fault/LConn2 -- Line2/LConn2 -- Line1/RConn2
  Fault/LConn1 -- Line2/LConn1 -- Line1/RConn1

== system OORT/Off-Line Analysis/Line 2 ==
  Fault : Subsystem
  Fault Selector : Subsystem
  Line1 : powerlib/Elements/Distributed Parameters Line  DialogController=POWERSYS.PowerSysDialog  SystemSampleTime=-1  Phases=3  Frequency=ff  Resistance=rr  Inductance=ll  Capacitance=cc  Length=length*faultLocation  x1=[0 4.37202236637398e-009 110076.231775724 -242919.997232943;3.63428122191995e-005 4.34324827738681e-009 113394.023147428 -241389.099530273;7.26856244383991e-005 4.31365890770207e-009 116690.529077365 -239812.890148216;0.000109028436657599 4.28325981160552e-009 119965.130771148 -238191.664960504;0.000145371248876798 4.2520566953784e-009 123217.213546082 -236525.728290888;0.000181714061095998 4.22005541622639e-009 126446.166946549 -234815.392856007]  x2=[0 5.10573142612213e-009 110362.200519469 -246631.419067912;3.63428122191995e-005 5.07018420151361e-009 113730.813344487 -245096.255114094;7.26856244383991e-005 5.03368524146458e-009 117078.077508108 -243515.08360255;0.000109028436657599 4.99624139727518e-009 120403.364688005 -241888.201338467;0.000145371248876798 4.95785969761187e-009 123706.050687201 -240215.913707496;0.000181714061095998 4.918547347188e-009 126985.515551233 -238498.534618431]  x3=[0 1.76988114683902e-011 166.597851371077 -992.559788072335;3.63428122191995e-005 1.78417362638266e-011 180.180769390775 -990.18415828643;7.26856244383991e-005 1.79813119476632e-011 193.72986528151 -987.622658851885;0.000109028436657599 1.81175123198409e-011 207.242595712658 -984.875770593398;0.000145371248876798 1.82503118138881e-011 220.716424179837 -981.944009135412;0.000181714061095998 1.83796855017194e-011 234.148821481038 -978.827924805327]  x4=[0 -5.53990670304512e-012 626.310821540122 -923.673067559427;3.63428122191995e-005 -5.73486715475771e-012 638.906810951093 -915.005610820616;7.26856244383991e-005 -5.92875110192906e-012 651.38286975777 -906.166396363844;0.000109028436657599 -6.12152215017654e-012 663.736656051683 -897.157083417521;0.000145371248876798 -6.31314411402221e-012 675.965850876405 -887.979363139617;0.000181714061095998 -6.50358102368531e-012 688.068158662848 -878.634958300214]  x5=0.000181714061095998  Measurements=None
  Line2 : powerlib/Elements/Distributed Parameters Line  DialogController=POWERSYS.PowerSysDialog  SystemSampleTime=-1  Phases=3  Frequency=ff  Resistance=rr  Inductance=ll  Capacitance=cc  Length=length*(1-faultLocation)  x1=[0 5.10573142612213e-009 110362.200519469 -246631.419067912;3.63428122191995e-005 5.07018420151361e-009 113730.813344487 -245096.255114094;7.26856244383991e-005 5.03368524146458e-009 117078.077508108 -243515.08360255;0.000109028436657599 4.99624139727518e-009 120403.364688005 -241888.201338467;0.000145371248876798 4.95785969761187e-009 123706.050687201 -240215.913707496;0.000181714061095998 4.918547347188e-009 126985.515551233 -238498.534618431]  x2=[0 5.82997759831409e-009 110739.990054586 -249234.046383737;3.63428122191995e-005 5.78954768315545e-009 114144.224688102 -247693.462256178;7.26856244383991e-005 5.74803099925317e-009 117527.033057867 -246106.383043422;0.000109028436657599 5.70543533979542e-009 120887.780169474 -244473.106659603;0.000145371248876798 5.66176870050723e-009 124225.835169682 -242793.939690626;0.000181714061095998 5.6170392781496e-009 127540.571464837 -241069.197336622]  x3=[0 1.44080502503912e-011 236.968633861882 -1005.53671745574;3.63428122191995e-005 1.45518794939418e-011 250.722737429789 -1002.19575558956;7.26856244383991e-005 1.46929771721508e-011 264.429777280586 -998.666669351373;0.000109028436657599 1.48313167992624e-011 278.087180435641 -994.950121193712;0.000145371248876798 1.49668724072404e-011 291.692383233736 -991.046808758018;0.000181714061095998 1.50996185506433e-011 305.242831812296 -986.957464743664]  x4=[0 -1.40022792260904e-012 557.75260993945 -935.152096479058;3.63428122191995e-005 -1.60721801226481e-012 570.512302263821 -927.422843372471;7.26856244383991e-005 -1.81390640748856e-012 583.164902467721 -919.51950168186;0.000109028436657599 -2.02025431034651e-012 595.708035503706 -911.443554960896;0.000145371248876798 -2.22622298681946e-012 608.139346872656 -903.19651916332;0.000181714061095998 -2.43177377407364e-012 620.456503065741 -894.779942358381]  x5=0.000181714061095998  Measurements=None
  Timer : powerlib_extras/Control  Blocks/Timer  DialogController=POWERSYS.PowerSysDialog  SystemSampleTime=-1  t=[0 faultTime]  e=[0 1 0 1 0 1]
  A1 : PMIOPort  Tag=PMCPort  Port=1  Side=Left
  B1 : PMIOPort  Tag=PMCPort  Port=2  Side=Left
  C1 : PMIOPort  Tag=PMCPort  Port=3  Side=Left
  A2 : PMIOPort  Tag=PMCPort  Port=4  Side=Right
  B2 : PMIOPort  Tag=PMCPort  Port=5  Side=Right
  C2 : PMIOPort  Tag=PMCPort  Port=6  Side=Right
  wires:
  Timer/1 -> Fault/5(Tfault)
  Fault Selector/4(faultG) -> Fault/4(faultG)
  Fault Selector/3(faultC) -> Fault/3(faultC)
  Fault Selector/2(faultB) -> Fault/2(faultB)
  Fault Selector/1(faultA) -> Fault/1(faultA)
  connections:
  Line2/RConn3 -- C2/RConn1
  Line2/RConn2 -- B2/RConn1
  Line2/RConn1 -- A2/RConn1
  C1/RConn1 -- Line1/LConn3
  B1/RConn1 -- Line1/LConn2
  A1/RConn1 -- Line1/LConn1
  Fault/LConn3 -- Line1/RConn3 -- Line2/LConn3
  Fault/LConn2 -- Line2/LConn2 -- Line1/RConn2
  Fault/LConn1 -- Line2/LConn1 -- Line1/RConn1
